simulink model "IPFC_Mathematicalmodel_MCHP"  (R2022a)
settings: Solver=ode8  StartTime=0.0  StopTime=10  RelTol=1e-3
values from neighbouring files (symbols this model uses):
  C = 4*680e-6    (= 0.00272)    [IPFC_Mathematicalmodel_MCHP_data.m]
  Ki_i = Kp_i/Tz_i    (= 7059.63868221)    [IPFC_Mathematicalmodel_MCHP_data.m]
  Ki_v = Kp_v/Tz_v    (= 30.6436278058)    [IPFC_Mathematicalmodel_MCHP_data.m]
  KiL = 1/Ibase    (= 0.042194092827)    [IPFC_Mathematicalmodel_MCHP_data.m]
  Kmul = Vpk_min/(2*Vbase)    (= 0.280927152318)    [IPFC_Mathematicalmodel_MCHP_data.m]
  Kp_i = Gci    (= 1.75558811362)    [IPFC_Mathematicalmodel_MCHP_data.m]
  Kp_v = Gcv    (= 4.87708483956)    [IPFC_Mathematicalmodel_MCHP_data.m]
  Kvin = 1/Vbase    (= 0.00220750551876)    [IPFC_Mathematicalmodel_MCHP_data.m]
  Kvo = 1/Vbase    (= 0.00220750551876)    [IPFC_Mathematicalmodel_MCHP_data.m]
  L1 = L    (= 0.0007)    [IPFC_Mathematicalmodel_MCHP_data.m]
  L2 = L    (= 0.0007)    [IPFC_Mathematicalmodel_MCHP_data.m]
  R = (Vout^2)/Po    (= 40.1111111111)    [IPFC_Mathematicalmodel_MCHP_data.m]
  Slope = (Vref-Vout_init)/T_rise    (= 547.8)    [IPFC_Mathematicalmodel_MCHP_data.m]
  Tsi = Isr / fsw    (= 1.5625e-05)    [IPFC_Mathematicalmodel_MCHP_data.m]
  Tsv = Osr / fsw    (= 0.00025)    [IPFC_Mathematicalmodel_MCHP_data.m]
  Vin_pk = Vin_rms*1.414    (= 325.22)    [IPFC_Mathematicalmodel_MCHP_data.m]
  Vin_rms = 230    [IPFC_Mathematicalmodel_MCHP_data.m]
libraries: slpidlib x3, spsSawtoothGeneratorLib x2, simulink x2, spsRMSLib x1, spsMeanLib x1
settings Model: Creator=I50990  LastModifiedBy=I50990

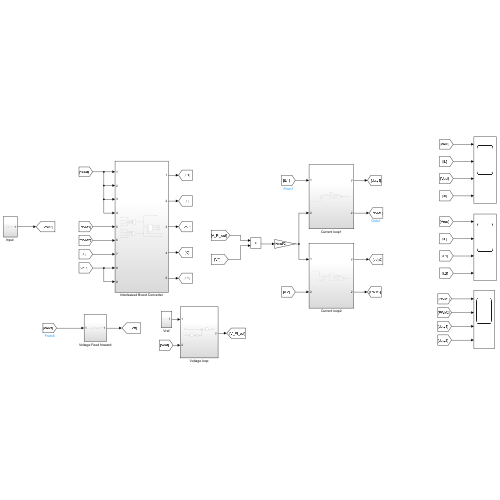
[thumbnail: Simulink's stored preview of the top-level diagram]
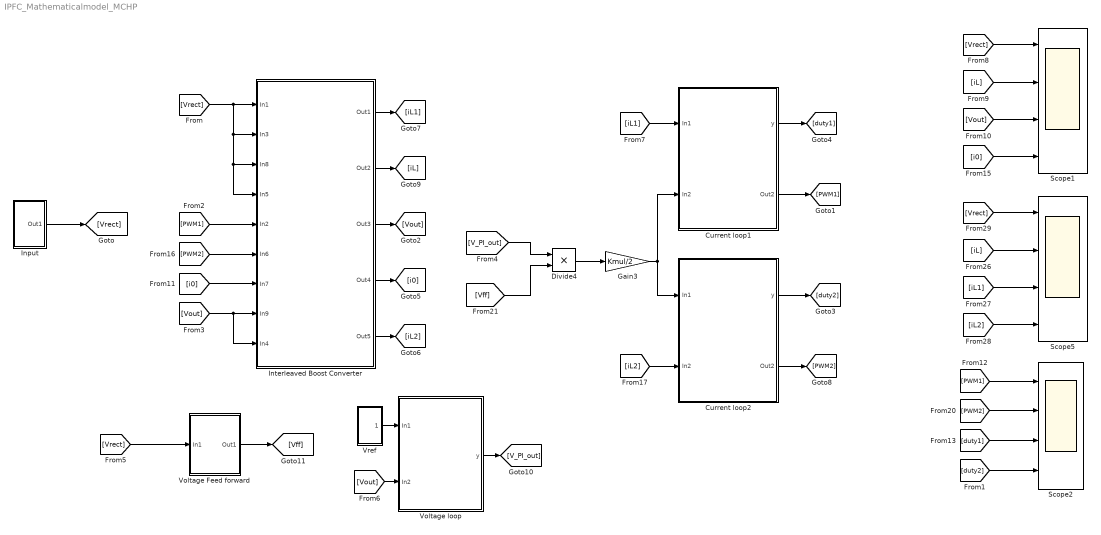
== system IPFC_Mathematicalmodel_MCHP ==
  Current loop1 : Subsystem
  Current loop2 : Subsystem
  Divide4 : Product  Inputs=**
  Gain3 : Gain  Gain=Kmul/2
  "Input " : Subsystem
  Interleaved Boost Converter : Subsystem
  Scope1 : Scope  NumInputPorts=4
  Scope2 : Scope  NumInputPorts=4
  Scope5 : Scope  NumInputPorts=4
  Voltage Feed forward : Subsystem
  Voltage loop : Subsystem
  Vref : Subsystem
  wires:
  Divide4/1 -> Gain3/1
  [Vrect] -> Scope1/1
  [iL] -> Scope1/2
  [Vout] -> Scope1/3
  [PWM1] -> Scope2/1
  [i0] -> Scope1/4
  "Input "/1(Out1) -> [Vrect]
  Gain3/1 -> Current loop1/2(In2), Current loop2/1(In1)
  [iL] -> Scope5/2
  [iL1] -> Scope5/3
  [iL2] -> Scope5/4
  [Vrect] -> Scope5/1
  [Vrect] -> Interleaved Boost Converter/4(In5), Interleaved Boost Converter/3(In8), Interleaved Boost Converter/2(In3), Interleaved Boost Converter/1(In1)
  [PWM1] -> Interleaved Boost Converter/5(In2)
  [Vout] -> Interleaved Boost Converter/9(In4), Interleaved Boost Converter/8(In9)
  [PWM2] -> Interleaved Boost Converter/6(In6)
  [i0] -> Interleaved Boost Converter/7(In7)
  Interleaved Boost Converter/1(Out1) -> [iL1]
  Interleaved Boost Converter/2(Out2) -> [iL]
  Interleaved Boost Converter/3(Out3) -> [Vout]
  Interleaved Boost Converter/4(Out4) -> [i0]
  Interleaved Boost Converter/5(Out5) -> [iL2]
  [V_PI_out] -> Divide4/1
  [Vff] -> Divide4/2
  [Vrect] -> Voltage Feed forward/1(In1)
  Voltage Feed forward/1(Out1) -> [Vff]
  Vref/1(Out1) -> Voltage loop/1(In1)
  [Vout] -> Voltage loop/2(In2)
  Voltage loop/1(y) -> [V_PI_out]
  [iL1] -> Current loop1/1(In1)
  Current loop1/1(y) -> [duty1]
  Current loop1/2(Out2) -> [PWM1]
  [iL2] -> Current loop2/2(In2)
  Current loop2/1(y) -> [duty2]
  Current loop2/2(Out2) -> [PWM2]
  [PWM2] -> Scope2/2
  [duty2] -> Scope2/4
  [duty1] -> Scope2/3

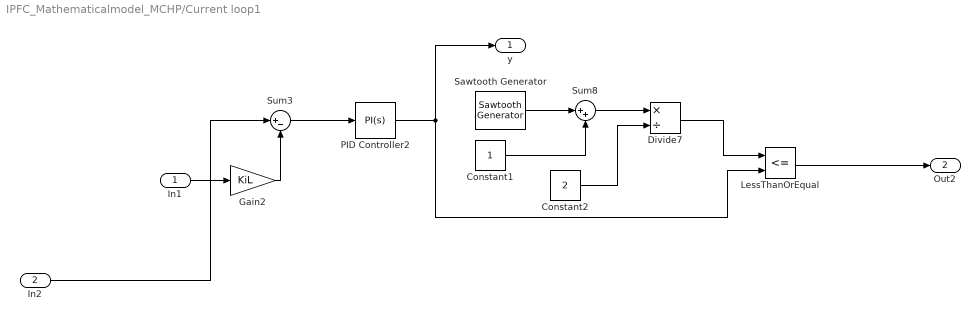
== system IPFC_Mathematicalmodel_MCHP/Current loop1 ==
  In1 : Inport
  In2 : Inport  Port=2
  Constant1 : Constant
  Constant2 : Constant  Value=2
  Divide7 : Product  Inputs=*/
  Gain2 : Gain  Gain=KiL
  LessThanOrEqual : RelationalOperator  Operator=<=  OutDataTypeStr=boolean  RndMeth=Simplest  InputSameDT=off
  PID Controller2 : slpidlib/PID Controller  Controller=PI  Form=Parallel  TimeDomain=Continuous-time  UseExternalTs=off  SampleTime=-1  IntegratorMethod=Forward Euler  FilterMethod=Forward Euler  ControllerParametersSource=internal  P=Kp_i  I=Ki_i  UseKiTs=off  D=0  N=100  UseFilter=on  TunerSelectOption=Transfer Function Based (PID Tuner App)  ZeroCross=off  InitialConditionSource=internal  InitialConditionForIntegrator=0  InitialConditionForFilter=0  DifferentiatorICPrevScaledInput=0  ExternalReset=none  TrackingMode=off  Kt=1  LimitOutput=on  SatLimitsSource=internal  UpperSaturationLimit=0.95  LowerSaturationLimit=0  LinearizeAsGain=on  AntiWindupMode=none  Kb=1  POutMin=[]  POutMax=[]  IOutMin=[]  IOutMax=[]  DOutMin=[]  DOutMax=[]  NOutMin=[]  NOutMax=[]  SumOutMin=[]  SumOutMax=[]  SaturationOutMin=[]  SaturationOutMax=[]  PParamMin=[]  PParamMax=[]  IParamMin=[]  IParamMax=[]  DParamMin=[]  DParamMax=[]  NParamMin=[]  NParamMax=[]  KbParamMin=[]  KbParamMax=[]  KtParamMin=[]  KtParamMax=[]  KbOutMin=[]  KbOutMax=[]  KtOutMin=[]  KtOutMax=[]  IntegratorOutMin=[]  IntegratorOutMax=[]  FilterOutMin=[]  FilterOutMax=[]  SumI1OutMin=[]  SumI1OutMax=[]  SumI2OutMin=[]  SumI2OutMax=[]  SumI3OutMin=[]  SumI3OutMax=[]  SumI4OutMin=[]  SumI4OutMax=[]  SumDOutMin=[]  SumDOutMax=[]  DifferentiatorOutMin=[]  DifferentiatorOutMax=[]  FilterDiffOutCoefMin=[]  FilterDiffOutCoefMax=[]  ReciprocalOutMin=[]  ReciprocalOutMax=[]  SumDenOutMin=[]  SumDenOutMax=[]  SumNumOutMin=[]  SumNumOutMax=[]  DivideOutMin=[]  DivideOutMax=[]  UdiffTsProdOutMin=[]  UdiffTsProdOutMax=[]  NTsProdOutMin=[]  NTsProdOutMax=[]  UintegralTsProdOutMin=[]  UintegralTsProdOutMax=[]  UngainTsProdOutMin=[]  UngainTsProdOutMax=[]  IntegratorContinuousStateAttributes=''  IntegratorStateMustResolveToSignalObject=off  IntegratorRTWStateStorageClass=Auto  FilterContinuousStateAttributes=''  FilterStateMustResolveToSignalObject=off  FilterRTWStateStorageClass=Auto  ParallelPVariant=InternalParameters  IdealPVariant=Disabled  IVariant=InternalParameters  DVariant=Disabled  IntegratorVariant=Continuous  SatVariant=Enabled  AWVariant=Passthrough  PCopyVariant=Disabled  TRVariant=Disabled  FdbkBlocksVariant=Forward  IdealPFdbkVariant=Disabled  SatFdbkVariant=Disabled  DerivativeFilterVariant=Disabled  NVariant=Disabled  NCopyVariant=Disabled_SignalSpec  FilterICVariant=Disabled  IntegratorICVariant=InternalICs  ExternalResetVariant=Disabled  TRSumVariant=Passthrough  SumFdbkVariant=Disabled  SumVariant=Sum_PI  TsampFilterVariant=InternalTs  TsampNgainVariant=Passthrough  TsampIntegralVariant=Passthrough  ExternalSaturationOutDataTypeStr=Inherit: Same as second input  aMode=0
  Sawtooth Generator : spsSawtoothGeneratorLib/Sawtooth Generator  Freq=fsw  Phase=0  Ts=Tsi/10
  Sum3 : Sum  Inputs=|+-
  Sum8 : Sum  Inputs=|++
  y : Outport
  Out2 : Outport  Port=2
  wires:
  Sum3/1 -> PID Controller2/1
  Gain2/1 -> Sum3/2
  Divide7/1 -> LessThanOrEqual/1
  PID Controller2/1 -> y/1, LessThanOrEqual/2
  Sum8/1 -> Divide7/1
  Constant1/1 -> Sum8/2
  Sawtooth Generator/1 -> Sum8/1
  Constant2/1 -> Divide7/2
  In1/1 -> Gain2/1
  LessThanOrEqual/1 -> Out2/1
  In2/1 -> Sum3/1

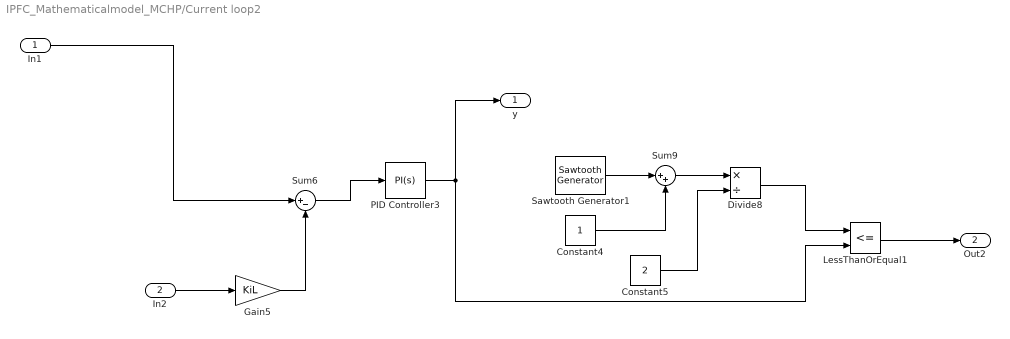
== system IPFC_Mathematicalmodel_MCHP/Current loop2 ==
  In1 : Inport
  In2 : Inport  Port=2
  Constant4 : Constant
  Constant5 : Constant  Value=2
  Divide8 : Product  Inputs=*/
  Gain5 : Gain  Gain=KiL
  LessThanOrEqual1 : RelationalOperator  Operator=<=  OutDataTypeStr=boolean  RndMeth=Simplest  InputSameDT=off
  PID Controller3 : slpidlib/PID Controller  Controller=PI  Form=Parallel  TimeDomain=Continuous-time  UseExternalTs=off  SampleTime=-1  IntegratorMethod=Forward Euler  FilterMethod=Forward Euler  ControllerParametersSource=internal  P=Kp_i  I=Ki_i  UseKiTs=off  D=0  N=100  UseFilter=on  TunerSelectOption=Transfer Function Based (PID Tuner App)  ZeroCross=off  InitialConditionSource=internal  InitialConditionForIntegrator=0  InitialConditionForFilter=0  DifferentiatorICPrevScaledInput=0  ExternalReset=none  TrackingMode=off  Kt=1  LimitOutput=on  SatLimitsSource=internal  UpperSaturationLimit=0.95  LowerSaturationLimit=0  LinearizeAsGain=on  AntiWindupMode=none  Kb=1  POutMin=[]  POutMax=[]  IOutMin=[]  IOutMax=[]  DOutMin=[]  DOutMax=[]  NOutMin=[]  NOutMax=[]  SumOutMin=[]  SumOutMax=[]  SaturationOutMin=[]  SaturationOutMax=[]  PParamMin=[]  PParamMax=[]  IParamMin=[]  IParamMax=[]  DParamMin=[]  DParamMax=[]  NParamMin=[]  NParamMax=[]  KbParamMin=[]  KbParamMax=[]  KtParamMin=[]  KtParamMax=[]  KbOutMin=[]  KbOutMax=[]  KtOutMin=[]  KtOutMax=[]  IntegratorOutMin=[]  IntegratorOutMax=[]  FilterOutMin=[]  FilterOutMax=[]  SumI1OutMin=[]  SumI1OutMax=[]  SumI2OutMin=[]  SumI2OutMax=[]  SumI3OutMin=[]  SumI3OutMax=[]  SumI4OutMin=[]  SumI4OutMax=[]  SumDOutMin=[]  SumDOutMax=[]  DifferentiatorOutMin=[]  DifferentiatorOutMax=[]  FilterDiffOutCoefMin=[]  FilterDiffOutCoefMax=[]  ReciprocalOutMin=[]  ReciprocalOutMax=[]  SumDenOutMin=[]  SumDenOutMax=[]  SumNumOutMin=[]  SumNumOutMax=[]  DivideOutMin=[]  DivideOutMax=[]  UdiffTsProdOutMin=[]  UdiffTsProdOutMax=[]  NTsProdOutMin=[]  NTsProdOutMax=[]  UintegralTsProdOutMin=[]  UintegralTsProdOutMax=[]  UngainTsProdOutMin=[]  UngainTsProdOutMax=[]  IntegratorContinuousStateAttributes=''  IntegratorStateMustResolveToSignalObject=off  IntegratorRTWStateStorageClass=Auto  FilterContinuousStateAttributes=''  FilterStateMustResolveToSignalObject=off  FilterRTWStateStorageClass=Auto  ParallelPVariant=InternalParameters  IdealPVariant=Disabled  IVariant=InternalParameters  DVariant=Disabled  IntegratorVariant=Continuous  SatVariant=Enabled  AWVariant=Passthrough  PCopyVariant=Disabled  TRVariant=Disabled  FdbkBlocksVariant=Forward  IdealPFdbkVariant=Disabled  SatFdbkVariant=Disabled  DerivativeFilterVariant=Disabled  NVariant=Disabled  NCopyVariant=Disabled_SignalSpec  FilterICVariant=Disabled  IntegratorICVariant=InternalICs  ExternalResetVariant=Disabled  TRSumVariant=Passthrough  SumFdbkVariant=Disabled  SumVariant=Sum_PI  TsampFilterVariant=InternalTs  TsampNgainVariant=Passthrough  TsampIntegralVariant=Passthrough  ExternalSaturationOutDataTypeStr=Inherit: Same as second input  aMode=0
  Sawtooth Generator1 : spsSawtoothGeneratorLib/Sawtooth Generator  Freq=fsw  Phase=180  Ts=Tsi/10
  Sum6 : Sum  Inputs=|+-
  Sum9 : Sum  Inputs=|++
  y : Outport
  Out2 : Outport  Port=2
  wires:
  Sum9/1 -> Divide8/1
  Gain5/1 -> Sum6/2
  Constant4/1 -> Sum9/2
  Divide8/1 -> LessThanOrEqual1/1
  Constant5/1 -> Divide8/2
  Sum6/1 -> PID Controller3/1
  PID Controller3/1 -> y/1, LessThanOrEqual1/2
  Sawtooth Generator1/1 -> Sum9/1
  LessThanOrEqual1/1 -> Out2/1
  In2/1 -> Gain5/1
  In1/1 -> Sum6/1

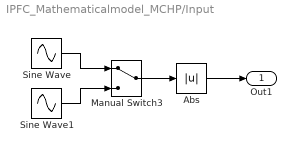
== system IPFC_Mathematicalmodel_MCHP/Input  ==
  Abs : Abs  SaturateOnIntegerOverflow=off
  Manual Switch3 : ManualSwitch
  Sine Wave : Sin  Amplitude=Vin_pk  Frequency=2*pi*50  SampleTime=0
  Sine Wave1 : Sin  Amplitude=Vin_pk/2  Frequency=2*pi*50  SampleTime=0
  Out1 : Outport
  wires:
  Sine Wave/1 -> Manual Switch3/1
  Manual Switch3/1 -> Abs/1
  Sine Wave1/1 -> Manual Switch3/2
  Abs/1 -> Out1/1

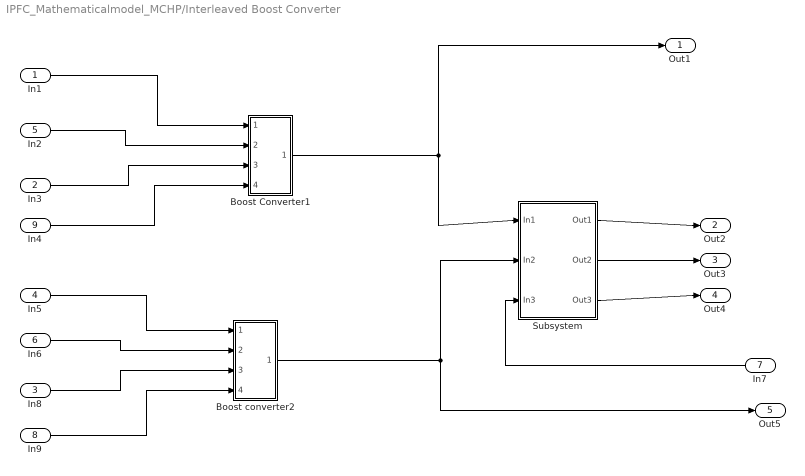
== system IPFC_Mathematicalmodel_MCHP/Interleaved Boost Converter ==
  In1 : Inport
  In3 : Inport  Port=2
  In8 : Inport  Port=3
  In5 : Inport  Port=4
  In2 : Inport  Port=5
  In6 : Inport  Port=6
  In7 : Inport  Port=7
  In9 : Inport  Port=8
  In4 : Inport  Port=9
  Boost Converter1 : Subsystem
  Boost converter2 : Subsystem
  Subsystem : Subsystem
  Out1 : Outport
  Out2 : Outport  Port=2
  Out3 : Outport  Port=3
  Out4 : Outport  Port=4
  Out5 : Outport  Port=5
  wires:
  In9/1 -> Boost converter2/4(In4)
  Boost converter2/1(Out1) -> Out5/1, Subsystem/2(In2)
  Boost Converter1/1(Out1) -> Out1/1, Subsystem/1(In1)
  In7/1 -> Subsystem/3(In3)
  In1/1 -> Boost Converter1/1(In1)
  In5/1 -> Boost converter2/1(In1)
  In8/1 -> Boost converter2/3(In3)
  In6/1 -> Boost converter2/2(In2)
  Subsystem/3(Out3) -> Out4/1
  Subsystem/1(Out1) -> Out2/1
  Subsystem/2(Out2) -> Out3/1
  In4/1 -> Boost Converter1/4(In4)
  In2/1 -> Boost Converter1/2(In2)
  In3/1 -> Boost Converter1/3(In3)

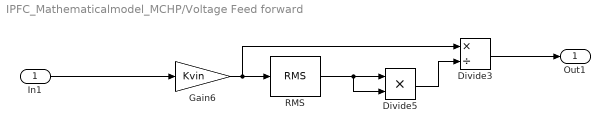
== system IPFC_Mathematicalmodel_MCHP/Voltage Feed forward ==
  In1 : Inport
  Divide3 : Product  Inputs=*/
  Divide5 : Product  Inputs=**
  Gain6 : Gain  Gain=Kvin
  RMS : spsRMSLib/RMS  TrueRMS=on  Freq=100  RMSInit=Vin_rms*Kvin  Ts=Tsi
  Out1 : Outport
  wires:
  Divide5/1 -> Divide3/2
  Gain6/1 -> Divide3/1, RMS/1
  RMS/1 -> Divide5/2, Divide5/1
  In1/1 -> Gain6/1
  Divide3/1 -> Out1/1

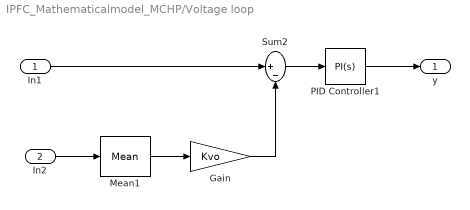
== system IPFC_Mathematicalmodel_MCHP/Voltage loop ==
  In1 : Inport
  In2 : Inport  Port=2
  Gain : Gain  Gain=Kvo
  Mean1 : spsMeanLib/Mean  Freq=100  Vinit=Vin_pk  Ts=Tsv
  PID Controller1 : slpidlib/PID Controller  Controller=PI  Form=Parallel  TimeDomain=Continuous-time  UseExternalTs=off  SampleTime=-1  IntegratorMethod=Forward Euler  FilterMethod=Forward Euler  ControllerParametersSource=internal  P=Kp_v  I=Ki_v  UseKiTs=off  D=0  N=100  UseFilter=on  TunerSelectOption=Transfer Function Based (PID Tuner App)  InitialConditionSource=internal  InitialConditionForIntegrator=0  InitialConditionForFilter=0  DifferentiatorICPrevScaledInput=0  ExternalReset=none  TrackingMode=off  Kt=1  LimitOutput=on  SatLimitsSource=internal  UpperSaturationLimit=1  LowerSaturationLimit=0  LinearizeAsGain=on  AntiWindupMode=none  Kb=1  POutMin=[]  POutMax=[]  IOutMin=[]  IOutMax=[]  DOutMin=[]  DOutMax=[]  NOutMin=[]  NOutMax=[]  SumOutMin=[]  SumOutMax=[]  SaturationOutMin=[]  SaturationOutMax=[]  PParamMin=[]  PParamMax=[]  IParamMin=[]  IParamMax=[]  DParamMin=[]  DParamMax=[]  NParamMin=[]  NParamMax=[]  KbParamMin=[]  KbParamMax=[]  KtParamMin=[]  KtParamMax=[]  KbOutMin=[]  KbOutMax=[]  KtOutMin=[]  KtOutMax=[]  IntegratorOutMin=[]  IntegratorOutMax=[]  FilterOutMin=[]  FilterOutMax=[]  SumI1OutMin=[]  SumI1OutMax=[]  SumI2OutMin=[]  SumI2OutMax=[]  SumI3OutMin=[]  SumI3OutMax=[]  SumI4OutMin=[]  SumI4OutMax=[]  SumDOutMin=[]  SumDOutMax=[]  DifferentiatorOutMin=[]  DifferentiatorOutMax=[]  FilterDiffOutCoefMin=[]  FilterDiffOutCoefMax=[]  ReciprocalOutMin=[]  ReciprocalOutMax=[]  SumDenOutMin=[]  SumDenOutMax=[]  SumNumOutMin=[]  SumNumOutMax=[]  DivideOutMin=[]  DivideOutMax=[]  UdiffTsProdOutMin=[]  UdiffTsProdOutMax=[]  NTsProdOutMin=[]  NTsProdOutMax=[]  UintegralTsProdOutMin=[]  UintegralTsProdOutMax=[]  UngainTsProdOutMin=[]  UngainTsProdOutMax=[]  IntegratorContinuousStateAttributes=''  IntegratorStateMustResolveToSignalObject=off  IntegratorRTWStateStorageClass=Auto  FilterContinuousStateAttributes=''  FilterStateMustResolveToSignalObject=off  FilterRTWStateStorageClass=Auto  ParallelPVariant=InternalParameters  IdealPVariant=Disabled  IVariant=InternalParameters  DVariant=Disabled  IntegratorVariant=Continuous  SatVariant=Enabled  AWVariant=Passthrough  PCopyVariant=Disabled  TRVariant=Disabled  FdbkBlocksVariant=Forward  IdealPFdbkVariant=Disabled  SatFdbkVariant=Disabled  DerivativeFilterVariant=Disabled  NVariant=Disabled  NCopyVariant=Disabled_SignalSpec  FilterICVariant=Disabled  IntegratorICVariant=InternalICs  ExternalResetVariant=Disabled  TRSumVariant=Passthrough  SumFdbkVariant=Disabled  SumVariant=Sum_PI  TsampFilterVariant=InternalTs  TsampNgainVariant=Passthrough  TsampIntegralVariant=Passthrough  ExternalSaturationOutDataTypeStr=Inherit: Same as second input  aMode=0
  Sum2 : Sum  Inputs=|+-
  y : Outport
  wires:
  In2/1 -> Mean1/1
  Gain/1 -> Sum2/2
  Mean1/1 -> Gain/1
  In1/1 -> Sum2/1
  Sum2/1 -> PID Controller1/1
  PID Controller1/1 -> y/1

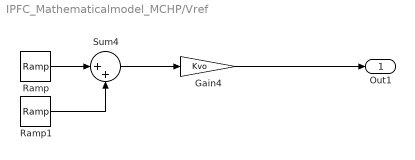
== system IPFC_Mathematicalmodel_MCHP/Vref ==
  Gain4 : Gain  Gain=Kvo
  Ramp : simulink/Sources/Ramp  slope=Slope  start=0  InitialOutput=Vin_pk
  Ramp1 : simulink/Sources/Ramp  slope=-Slope  start=T_rise  InitialOutput=0
  Sum4 : Sum  Inputs=|++
  Out1 : Outport
  wires:
  Ramp/1 -> Sum4/1
  Sum4/1 -> Gain4/1
  Ramp1/1 -> Sum4/2
  Gain4/1 -> Out1/1

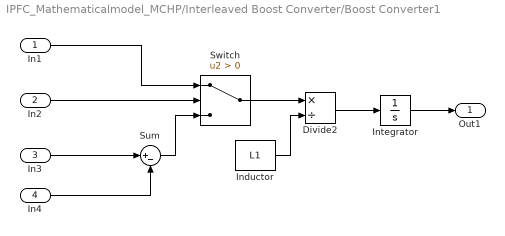
== system IPFC_Mathematicalmodel_MCHP/Interleaved Boost Converter/Boost Converter1 ==
  In1 : Inport
  In2 : Inport  Port=2
  In3 : Inport  Port=3
  In4 : Inport  Port=4
  Divide2 : Product  Inputs=*/
  Inductor : Constant  Value=L1  SampleTime=Tsi
  Integrator : Integrator
  Sum : Sum  Inputs=|+-
  Switch : Switch  Criteria=u2 > Threshold  SaturateOnIntegerOverflow=off  InputSameDT=off
  Out1 : Outport
  wires:
  In3/1 -> Sum/1
  Sum/1 -> Switch/3
  Integrator/1 -> Out1/1
  Inductor/1 -> Divide2/2
  Switch/1 -> Divide2/1
  Divide2/1 -> Integrator/1
  In2/1 -> Switch/2
  In1/1 -> Switch/1
  In4/1 -> Sum/2

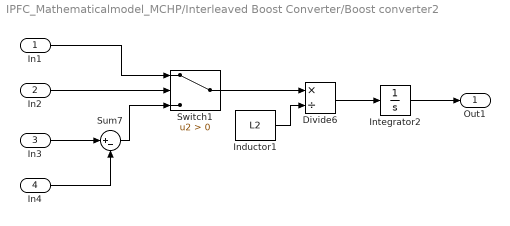
== system IPFC_Mathematicalmodel_MCHP/Interleaved Boost Converter/Boost converter2 ==
  In1 : Inport
  In2 : Inport  Port=2
  In3 : Inport  Port=3
  In4 : Inport  Port=4
  Divide6 : Product  Inputs=*/
  Inductor1 : Constant  Value=L2  SampleTime=Tsi
  Integrator2 : Integrator
  Sum7 : Sum  Inputs=|+-
  Switch1 : Switch  Criteria=u2 > Threshold  SaturateOnIntegerOverflow=off  InputSameDT=off
  Out1 : Outport
  wires:
  Switch1/1 -> Divide6/1
  In4/1 -> Sum7/2
  In3/1 -> Sum7/1
  Divide6/1 -> Integrator2/1
  Inductor1/1 -> Divide6/2
  Sum7/1 -> Switch1/3
  Integrator2/1 -> Out1/1
  In1/1 -> Switch1/1
  In2/1 -> Switch1/2

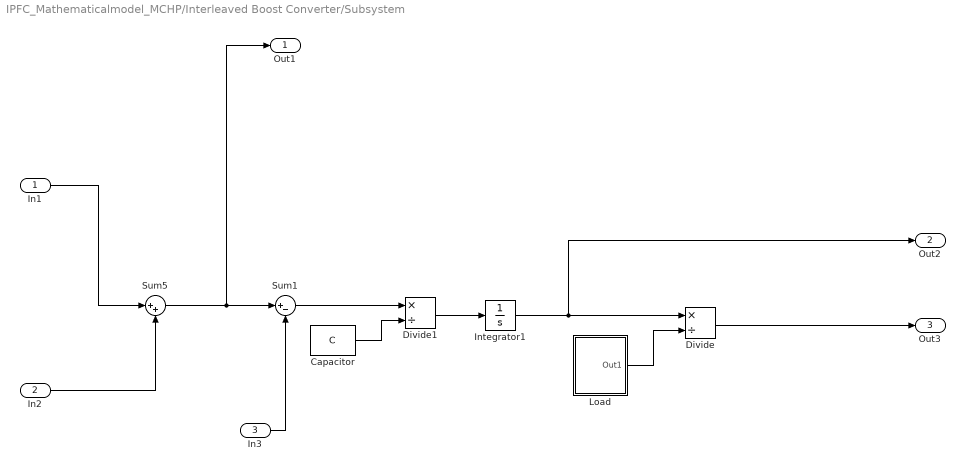
== system IPFC_Mathematicalmodel_MCHP/Interleaved Boost Converter/Subsystem ==
  In1 : Inport
  In2 : Inport  Port=2
  In3 : Inport  Port=3
  Capacitor : Constant  Value=C  SampleTime=Tsi
  Divide : Product  Inputs=*/
  Divide1 : Product  Inputs=*/
  Integrator1 : Integrator  InitialCondition=Vin_pk
  Load : Subsystem
  Sum1 : Sum  Inputs=|+-
  Sum5 : Sum  Inputs=|++
  Out1 : Outport
  Out2 : Outport  Port=2
  Out3 : Outport  Port=3
  wires:
  Integrator1/1 -> Out2/1, Divide/1
  In2/1 -> Sum5/2
  Sum1/1 -> Divide1/1
  In1/1 -> Sum5/1
  Divide1/1 -> Integrator1/1
  Capacitor/1 -> Divide1/2
  Sum5/1 -> Out1/1, Sum1/1
  Load/1(Out1) -> Divide/2
  Divide/1 -> Out3/1
  In3/1 -> Sum1/2

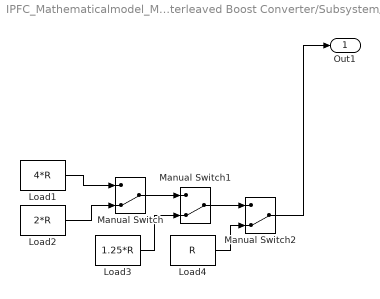
== system IPFC_Mathematicalmodel_MCHP/Interleaved Boost Converter/Subsystem/Load ==
  Load1 : Constant  Value=4*R  SampleTime=Tsi
  Load2 : Constant  Value=2*R  SampleTime=Tsi
  Load3 : Constant  Value=1.25*R  SampleTime=Tsi
  Load4 : Constant  Value=R  SampleTime=Tsi
  Manual Switch : ManualSwitch  CurrentSetting=0
  Manual Switch1 : ManualSwitch  CurrentSetting=0
  Manual Switch2 : ManualSwitch  CurrentSetting=0
  Out1 : Outport
  wires:
  Load3/1 -> Manual Switch1/2
  Load2/1 -> Manual Switch/2
  Manual Switch1/1 -> Manual Switch2/1
  Load4/1 -> Manual Switch2/2
  Manual Switch2/1 -> Out1/1
  Manual Switch/1 -> Manual Switch1/1
  Load1/1 -> Manual Switch/1
